simulink library "mode_selection"  (R2016b)
settings: Solver=VariableStepAuto  StartTime=0.0  StopTime=10.0  RelTol=1e-3
undefined symbols (not defined in the file or in its folder): fsw_params
settings Model: Creator=taylorreynolds  LastModifiedBy=Taylor

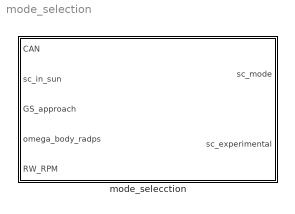
== system mode_selection ==
  mode_selecction : Subsystem

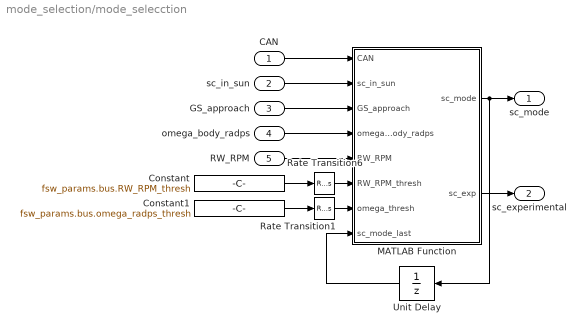
== system mode_selection/mode_selecction ==
  CAN : Inport
  sc_in_sun : Inport  Port=2
  GS_approach : Inport  Port=3
  omega_body_radps : Inport  Port=4
  RW_RPM : Inport  Port=5
  Constant : Constant  Value=fsw_params.bus.RW_RPM_thresh
  Constant1 : Constant  Value=fsw_params.bus.omega_radps_thresh
  MATLAB Function : MATLAB Function  TreatAsAtomicUnit=on
  Rate Transition1 : RateTransition  OutPortSampleTime=fsw_params.sample_time_s
  Rate Transition6 : RateTransition  OutPortSampleTime=fsw_params.sample_time_s
  Unit Delay : UnitDelay  SampleTime=-1
  sc_mode : Outport
  sc_experimental : Outport  Port=2
  wires:
  GS_approach/1 -> MATLAB Function/3(GS_approach)
  Unit Delay/1 -> MATLAB Function/8(sc_mode_last)
  MATLAB Function/2(sc_exp) -> sc_experimental/1
  Rate Transition1/1 -> MATLAB Function/7(omega_thresh)
  Rate Transition6/1 -> MATLAB Function/6(RW_RPM_thresh)
  CAN/1 -> MATLAB Function/1(CAN)
  RW_RPM/1 -> MATLAB Function/5(RW_RPM)
  sc_in_sun/1 -> MATLAB Function/2(sc_in_sun)
  omega_body_radps/1 -> MATLAB Function/4(omega_body_radps)
  MATLAB Function/1(sc_mode) -> Unit Delay/1, sc_mode/1
  Constant/1 -> Rate Transition6/1
  Constant1/1 -> Rate Transition1/1

== matlab function mode_selection/mode_selecction/MATLAB Function ==
  data: CAN input; sc_in_sun input; GS_approach input; omega_body_radps input; sc_mode output; RW_RPM input; RW_RPM_thresh input; omega_thresh input; sc_exp output; sc_mode_last input
function [sc_mode,sc_exp] = fcn(CAN,sc_in_sun,GS_approach,omega_body_radps,RW_RPM,RW_RPM_thresh,omega_thresh,sc_mode_last)

% Main FSW Mode Selector
%   UW HuskySat-1, ADCS Team
%   Last Updated: T. Reynolds 11.9.17

% Chooses control mode based on sensor and actuator data.
%   mode_logic.bdot             = 1;
%   mode_logic.desat_eclipse    = 2;
%   mode_logic.point            = 3;
%       point.velocity          = 31;
%       point.ground            = 32;
%       point.MPC               = 33;
%   mode_logic.low_power        = 4;
%
% ----- INPUTS -----
%
% CAN - Data coming over the CAN bus. Type: 6x1 double. Parsed according to:
%
%   CAN(1) == Override the autonomous mode selection and command the mode
%               corresponding to this number. Set to 0 if the autonomous 
%               selection is to go ahead.
%   CAN(2) == Reboot just occured. Value: 0,1. Want this flipped to 1 upon
%               exiting a detumble, and flipped to 0 after [60] seconds.
%   CAN(3) == Go ahead for the pointing mode. Value: 0,1. One means the s/c
%               is go for pointing of any kind.
%   CAN(4) == Go ahead for COM2 and GS pointing. Value: 0,1. One means that
%               the COM2 system will be booted on the next flyover.
%   CAN(5) == PPT On. Value: 0,1. Zero implies PPT is off and will not fire
%               on the next sync cycle.
%   CAN(6) == Go ahead for ADCS experimental control. Value: 0,1. One
%               means ADCS has the go ahead.
%   CAN(7) == Type of pointing for experimental control. To be passed to the
%               MPC parser for target generation.
%
% sc_in_sun: - Tells us if the s/c is in eclipse. Type: 1x1 boolean.
%
% GS_appraoch: - Tells us if the ground station is approaching based on
%                   reorientation criteria. Type: 1x1 boolean.
%
% omega_body_radps - S/c bus angular velocity. Type: 3x1 double.
%
% RW_RPM - reaction wheel RPM values. Type 3x1 double.
%
% RW_RPM_thresh - Upper and lower thresholds for desaturation. Type: 2x1
%                   int. Parsed according to:
%   RW_RPM_thresh(1) == lower threshold, below which desat cedes control.
%   RW_RPM_thresh(2) == upper threshold, above which desat is triggered.
%
% omega_thresh - Upper and lower thresholds for detumble. Type: 2x1 int.
%                   Parsed according to:
%   omega_thresh(1) == lower threshold, below which the s/c is "detumbled"
%   omega_thresh(2) == upper threshold, above which detumble is triggered
%
% sc_mode_old - Previous spacecraft state, used to test exit conditions for
%                   each mode.
%
%
% ----- OUTPUTS -----
%
% sc_mode - Spacecraft state determined. Type: double.
%
% sc_exp - Extra state corresponding to what type of experimental control
%           is engaged. Only nonzero if sc_mode == 33.
%
% ----------------------------------------------------------------------- %

% Default to bdot and no experimental control
sc_mode     = 1;
sc_exp      = 0;

if( CAN(1) == 0 )
    
    % Check for bdot condition
    if( norm(omega_body_radps,inf) >= omega_thresh(1) )
        sc_mode     = 1;
        % If Bdot is triggered, return immediately since control has high 
        % priority and control will be handed off.
        return;
    else
        % If body rate is below upper thresh, but not below lower thresh,
        % then stay in bdot mode.
        sc_mode     = sc_mode_last;
    end
    
    % If we're in Bdot mode, require that body rates drop below thresh
    % before looking at other modes.
    if( norm(omega_body_radps,inf) <= omega_thresh(2) )
        
        % Check for low power condition or recent boot up
        if( CAN(2) == 1 )
            % If reboot just occured and we are not tumbling, enter low
            % power/estimate mode.
            sc_mode     = 4;
            return;
        else
            % If CAN does not say to stay in low power/estimate mode, then
            % default to last known mode until someone downstream takes
            % over.
            sc_mode     = sc_mode_last;
        end
        
        % Check exit condition for low power/estimation. THIS EXIT
        % CONDITION NEEDS WORK. THINK ABOUT HOW TO IMPLEMENT. EVERYTHING
        % BELOW THIS POINT HAS NOT BEEN THOUGHT OUT ENTIRELY.
        if( CAN(2) == 0 )
            
            % Check for desat conditions. This is for dedicated desat
            % event. 
            if( ~sc_in_sun && (norm(RW_RPM,inf)>=RW_RPM_thresh(2)) )
                if( CAN(5) == 0 )
                    sc_mode     = 2;
                else
                    % How to tell the s/c that we want to do deSat and the
                    % PPT should shut off?
                end
            end
            
            % Check for pointing condition from CAN
            if( CAN(3) == 1 )
                % Default to velocity pointing mode
                sc_mode     = 31;
                
                % Check to see if entering GS range, not in eclipse and 
                % COM2 system will be activated.
                if( GS_approach && sc_in_sun && (CAN(4)==1) )
                    sc_mode  = 32;
                end
                
                % Check for permission to enter experimental mode
                if( sc_in_sun && CAN(6) == 1 )
                    % Set experimental mode to the commanded value for target state
                    % generation.
                    if( GS_approach && CAN(7) == 1)
                        sc_exp  = 1;
                    elseif( CAN(7) == 2 )
                        sc_exp  = 2;
                    end
                        
                end
                
            end
            
        end
        
    end
    
    
% If signal received to override the autonomous mode selection, set mode 
% based on CAN(1) value.
elseif( CAN(1) ~= 0 )
    
    sc_mode = CAN(1);
    
end
